simulink model "transpose_core"  (R2016b)
settings: Solver=VariableStepAuto  StartTime=0.0  StopTime=512 * 64 * 3  RelTol=1e-3
model workspace (MAT data in the model file):
  dstin = [0 168430081 168430082 168430083 168430084 168430085 168430086 168430087 168430088 168430089 168430090 168430091 ... (33 elements, 1x33)]
  simin = [1 2 3 4 5 6 7 8 9 10 11 12 ... (294912 elements, 98304x3)]
libraries: xbsIndex_r4 x31
(part 2 of 2)

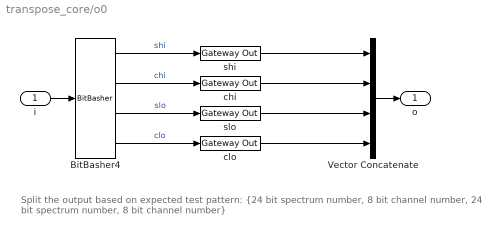
== system transpose_core/o0 ==
  note: Split the output based on expected test pattern:
      | {24 bit spectrum number, 8 bit channel number, 24 bit spectrum number, 8 bit channel number}
  i : Inport
  BitBasher4 : xbsIndex_r4/BitBasher  bitexpr=|  display_expr=off  sr_1=shi  arith_type1=Unsigned  bin_pt1=0  sr_2=chi  arith_type2=Unsigned  bin_pt2=0  sr_3=slo  arith_type3=Unsigned  bin_pt3=0  sr_4=clo  arith_type4=Unsigned  bin_pt4=0  dbl_ovrd=off  block_type=bitbasher
      | shi={o[63:40]}
      | chi={o[39:32]}
      | slo={o[31:8]}
      | clo={o[7:0]}
  Vector Concatenate : Concatenate  NumInputs=4
  chi : xbsIndex_r4/Gateway Out  inherit_from_input=off  hdl_port=off  rows=1  columns=1  UseAsDAC=off  DACChannel='1'  interface=None  automatic_assignment=on  address_offset=hex2dec('00')  intf_name=''  intf_description=''  timing_constraint=None  locs_specified=off  LOCs={}  io_standard={}  block_type=gatewayout
  clo : xbsIndex_r4/Gateway Out  inherit_from_input=off  hdl_port=off  rows=1  columns=1  UseAsDAC=off  DACChannel='1'  interface=None  automatic_assignment=on  address_offset=hex2dec('00')  intf_name=''  intf_description=''  timing_constraint=None  locs_specified=off  LOCs={}  io_standard={}  block_type=gatewayout
  shi : xbsIndex_r4/Gateway Out  inherit_from_input=off  hdl_port=off  rows=1  columns=1  UseAsDAC=off  DACChannel='1'  interface=None  automatic_assignment=on  address_offset=hex2dec('00')  intf_name=''  intf_description=''  timing_constraint=None  locs_specified=off  LOCs={}  io_standard={}  block_type=gatewayout
  slo : xbsIndex_r4/Gateway Out  inherit_from_input=off  hdl_port=off  rows=1  columns=1  UseAsDAC=off  DACChannel='1'  interface=None  automatic_assignment=on  address_offset=hex2dec('00')  intf_name=''  intf_description=''  timing_constraint=None  locs_specified=off  LOCs={}  io_standard={}  block_type=gatewayout
  o : Outport
  wires:
  BitBasher4/1 -> shi/1  "shi"
  BitBasher4/2 -> chi/1  "chi"
  i/1 -> BitBasher4/1
  Vector Concatenate/1 -> o/1
  BitBasher4/3 -> slo/1  "slo"
  BitBasher4/4 -> clo/1  "clo"
  shi/1 -> Vector Concatenate/1
  chi/1 -> Vector Concatenate/2
  slo/1 -> Vector Concatenate/3
  clo/1 -> Vector Concatenate/4

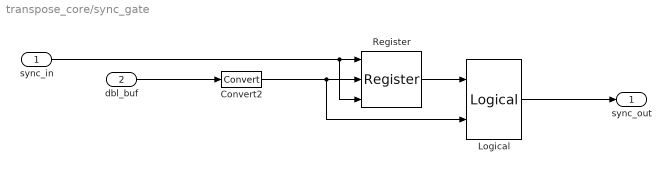
== system transpose_core/sync_gate ==
  sync_in : Inport
  dbl_buf : Inport  Port=2
  Convert2 : xbsIndex_r4/Convert  gui_display_data_type=Boolean  arith_type=Boolean  n_bits=16  bin_pt=14  float_type=Single  exp_bits=8  fraction_bits=24  quantization=Truncate  overflow=Wrap  en=off  latency=0  pipeline=off  dbl_ovrd=off  block_type=convert
  Logical : xbsIndex_r4/Logical  logical_function=AND  inputs=2  en=off  latency=0  precision=Full  arith_type=Unsigned  n_bits=16  bin_pt=0  align_bp=on  dbl_ovrd=off  block_type=logical
  Register : xbsIndex_r4/Register  init=0  rst=on  en=on  dbl_ovrd=off  block_type=register
  sync_out : Outport
  wires:
  Logical/1 -> sync_out/1
  Convert2/1 -> Logical/2, Register/2
  dbl_buf/1 -> Convert2/1
  Register/1 -> Logical/1
  sync_in/1 -> Register/1, Register/3
